simulink model "SHY4_S2"  (R2023a)
settings: Solver=VariableStepAuto  StartTime=0.0  StopTime=1000  RelTol=1e-3
values from neighbouring files (symbols this model uses):
  coolant_initial_temperature = 293.15    [cathode_subsystem_parameters.m]    (also in thermal_subsystem_parameters.m)
  coolant_tube_D = 0.05    [cathode_subsystem_parameters.m]    (also in thermal_subsystem_parameters.m)
  Hydrowell_VTS =     [Hydrowell_values_VLV.mat]
undefined symbols (not defined in the file or in its folder): sigbuilder_block, stack
libraries: fl_lib x135, nesl_utility x104, SimscapeFluids_lib x15, slpidlib x5, simulink x1
(part 3 of 8)

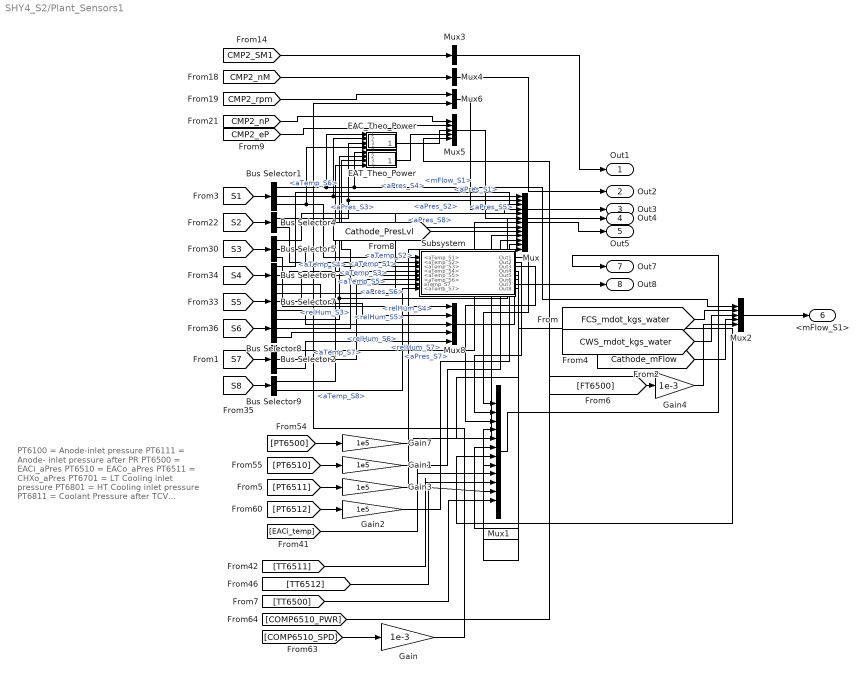
== system SHY4_S2/Plant_Sensors1 ==
  note: PT6100 = Anode-inlet pressure
      | PT6111 = Anode- inlet pressure after PR
      | PT6500 = EACi_aPres
      | PT6510 = EACo_aPres
      | PT6511 = CHXo_aPres
      | PT6701 = LT Cooling inlet pressure
      | PT6801 = HT Cooling inlet pressure
      | PT6811 = Coolant Pressure after TCV
      | PT6114 = FCS H2 inlet pressure
      | PT6512 = FCS O2 inlet Pressure
      | PT6812 = FCS Coolant inlet pressure
      |
      | TT6100 = Anode- inlet Temperature
      | TT6111 = Anode- after Temperature
      | TT6500 = EACi_Temp
      | TT6510 = EACo_Temp
      | TT6701 = LT Cooling inlet Temperature
      | TT6801 = HT Cooling inlet Temperature
      | TT6811 = Coolant Temperature after TCV
      | TT6114 = FCS H2 inlet Temperature
      | TT6512 = FCS O2 inlet Temperature
      | TT6812 = FCS Coolant inlet Temperature
  Bus Selector1 : BusSelector  OutputSignals=mFlow_S1,aPres_S1,aTemp_S1
  Bus Selector2 : BusSelector  OutputSignals=aPres_S7,aTemp_S7,relHum_S7
  Bus Selector4 : BusSelector  OutputSignals=aPres_S2,aTemp_S2
  Bus Selector5 : BusSelector  OutputSignals=aPres_S3,aTemp_S3,relHum_S3
  Bus Selector6 : BusSelector  OutputSignals=aPres_S4,aTemp_S4,relHum_S4
  Bus Selector7 : BusSelector  OutputSignals=aPres_S5,aTemp_S5,relHum_S5
  Bus Selector8 : BusSelector  OutputSignals=aPres_S6,aTemp_S6,relHum_S6
  Bus Selector9 : BusSelector  OutputSignals=aPres_S8,aTemp_S8
  EAC_Theo_Power : Subsystem
  EAT_Theo_Power : Subsystem
  Gain : Gain  Gain=1e-3
  Gain{1..3,7} (4 alike) : Gain  Gain=1e5
  Gain4 : Gain  Gain=1e-3
  Mux : Mux  Inputs=13
  Mux1 : Mux  Inputs=12
  Mux2 : Mux  Inputs=5
  Mux3 : Mux  Inputs=1
  Mux4 : Mux  Inputs=1
  Mux5 : Mux  Inputs=5
  Mux6 : Mux  Inputs=2
  Mux8 : Mux  Inputs=5
  Subsystem : Subsystem
  Out1 : Outport
  Out2 : Outport  Port=2
  Out3 : Outport  Port=3
  Out4 : Outport  Port=4
  Out5 : Outport  Port=5
  <mFlow_S1> : Outport  Port=6
  Out7 : Outport  Port=7
  Out8 : Outport  Port=8
  wires:
  [CMP2_eP] -> Mux5/2
  [CMP2_nP] -> Mux5/1
  Mux3/1 -> Out1/1
  [S8] -> Bus Selector9/1
  [CMP2_SM1] -> Mux3/1
  Bus Selector7/3 -> Mux8/3  "<relHum_S5>"
  Bus Selector9/1 -> EAT_Theo_Power/4(<aPres_S7>), Mux/8  "<aPres_S8>"
  Bus Selector4/1 -> EAC_Theo_Power/3(<aPres_S2>), Mux/2  "<aPres_S2>"
  [CMP2_rpm] -> Mux6/1
  [CMP2_nM] -> Mux4/1
  Bus Selector6/1 -> Mux/4  "<aPres_S4>"
  [S5] -> Bus Selector7/1
  Mux/1 -> Out5/1
  Bus Selector5/3 -> Mux8/1  "<relHum_S3>"
  Bus Selector5/1 -> Mux/3  "<aPres_S3>"
  [S4] -> Bus Selector6/1
  Mux6/1 -> Out3/1
  [S3] -> Bus Selector5/1
  Bus Selector1/1 -> Mux2/1, EAT_Theo_Power/1(<mFlow_S1>), EAC_Theo_Power/1(<mFlow_S1>)  "<mFlow_S1>"
  Bus Selector7/1 -> Mux/5  "<aPres_S5>"
  Bus Selector8/1 -> EAT_Theo_Power/2(<aPres_S6>), Mux/6  "<aPres_S6>"
  [S1] -> Bus Selector1/1
  [Cathode_PresLvl] -> Mux/9
  Mux5/1 -> Out4/1
  Bus Selector6/3 -> Mux8/2  "<relHum_S4>"
  Bus Selector8/3 -> Mux8/4  "<relHum_S6>"
  [S6] -> Bus Selector8/1
  Bus Selector1/2 -> Mux/1, EAC_Theo_Power/2(<aPres_S1>)  "<aPres_S1>"
  [S2] -> Bus Selector4/1
  Mux4/1 -> Out2/1
  Mux1/1 -> Out7/1
  Mux8/1 -> Out8/1
  Bus Selector1/3 -> EAC_Theo_Power/4(<aTemp_S1>), Subsystem/1(<aTemp_S1>)  "<aTemp_S1>"
  Bus Selector4/2 -> Subsystem/2(<aTemp_S2>)  "<aTemp_S2>"
  Bus Selector5/2 -> Subsystem/3(<aTemp_S3>)  "<aTemp_S3>"
  Bus Selector6/2 -> Subsystem/4(<aTemp_S4>)  "<aTemp_S4>"
  Bus Selector7/2 -> Subsystem/5(<aTemp_S5>)  "<aTemp_S5>"
  Bus Selector8/2 -> EAT_Theo_Power/3(<aTemp_S6>), Subsystem/6(<aTemp_S6>)  "<aTemp_S6>"
  Bus Selector9/2 -> Subsystem/8(<aTemp_S7>)  "<aTemp_S8>"
  Subsystem/1(Out1) -> Mux1/1
  Subsystem/2(Out2) -> Mux1/2
  Subsystem/3(Out3) -> Mux1/3
  Subsystem/4(Out4) -> Mux1/4
  Subsystem/5(Out5) -> Mux1/5
  Subsystem/6(Out6) -> Mux1/6
  Subsystem/7(Out7) -> Mux1/7
  EAC_Theo_Power/1(Out1) -> Mux5/3
  EAT_Theo_Power/1(Out1) -> Mux5/4
  [S7] -> Bus Selector2/1
  Bus Selector2/2 -> Subsystem/7(aTemp_S7)  "<aTemp_S7>"
  Subsystem/8(Out8) -> Mux1/8
  Bus Selector2/1 -> Mux/7  "<aPres_S7>"
  Bus Selector2/3 -> Mux8/5  "<relHum_S7>"
  [FCS_mdot_kgs_water] -> Mux2/2
  Mux2/1 -> <mFlow_S1>/1
  [Cathode_mFlow] -> Mux2/4
  [CWS_mdot_kgs_water] -> Mux2/3
  Gain1/1 -> Mux/11
  [COMP6510_SPD] -> Gain/1
  Gain2/1 -> Mux/12
  [PT6500] -> Gain7/1
  [EACi_temp] -> Mux1/9
  [TT6512] -> Mux1/11
  [PT6512] -> Gain2/1
  [TT6500] -> Mux1/12
  [TT6511] -> Mux1/10
  [COMP6510_PWR] -> Mux5/5
  [PT6510] -> Gain1/1
  Gain7/1 -> Mux/10
  Gain/1 -> Mux6/2
  [PT6511] -> Gain3/1
  Gain3/1 -> Mux/13
  [FT6500] -> Gain4/1
  Gain4/1 -> Mux2/5

== system SHY4_S2/Subsystem ==
  <aTemp_S4> : Inport
  Constant : Constant  Value=273.15
  Minus : Sum  Inputs=+-
  Out1 : Outport
  wires:
  Constant/1 -> Minus/2
  <aTemp_S4>/1 -> Minus/1
  Minus/1 -> Out1/1

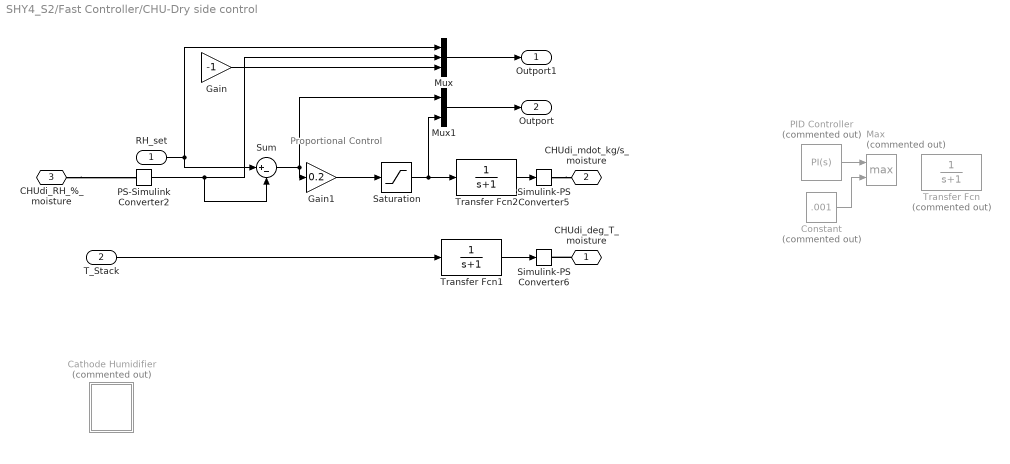
== system SHY4_S2/Fast Controller/CHU-Dry side control ==
  note: Proportional Control
  RH_set : Inport
  T_Stack : Inport  Port=2
  Cathode Humidifier : Subsystem  Tag=PublishSubsystem  Commented=on
  Constant : Constant  Commented=on  Value=.001
  Gain : Gain  Gain=-1
  Gain1 : Gain  Gain=0.2
  Max : MinMax  Commented=on  Function=max  Inputs=2
  Mux : Mux  Inputs=3
  Mux1 : Mux  Inputs=2
  PID Controller : slpidlib/PID Controller  Commented=on  Controller=PI  Form=Parallel  TimeDomain=Continuous-time  UseExternalTs=off  SampleTime=-1  IntegratorMethod=Forward Euler  FilterMethod=Forward Euler  ControllerParametersSource=internal  P=1  I=1  UseKiTs=off  D=0  N=100  UseFilter=on  TunerSelectOption=Transfer Function Based (PID Tuner App)  InitialConditionSource=internal  InitialConditionForIntegrator=0  InitialConditionForFilter=0  DifferentiatorICPrevScaledInput=0  ExternalReset=none  TrackingMode=off  Kt=1  LimitOutput=off  SatLimitsSource=internal  UpperSaturationLimit=inf  LowerSaturationLimit=-inf  LinearizeAsGain=on  AntiWindupMode=none  Kb=1  LimitIntegrator=off  UpperIntegratorSaturationLimit=inf  LowerIntegratorSaturationLimit=-inf  POutMin=[]  POutMax=[]  IOutMin=[]  IOutMax=[]  DOutMin=[]  DOutMax=[]  NOutMin=[]  NOutMax=[]  SumOutMin=[]  SumOutMax=[]  SaturationOutMin=[]  SaturationOutMax=[]  PParamMin=[]  PParamMax=[]  IParamMin=[]  IParamMax=[]  DParamMin=[]  DParamMax=[]  NParamMin=[]  NParamMax=[]  KbParamMin=[]  KbParamMax=[]  KtParamMin=[]  KtParamMax=[]  KbOutMin=[]  KbOutMax=[]  KtOutMin=[]  KtOutMax=[]  IntegratorOutMin=[]  IntegratorOutMax=[]  FilterOutMin=[]  FilterOutMax=[]  SumI1OutMin=[]  SumI1OutMax=[]  SumI2OutMin=[]  SumI2OutMax=[]  SumI3OutMin=[]  SumI3OutMax=[]  SumI4OutMin=[]  SumI4OutMax=[]  SumDOutMin=[]  SumDOutMax=[]  DifferentiatorOutMin=[]  DifferentiatorOutMax=[]  FilterDiffOutCoefMin=[]  FilterDiffOutCoefMax=[]  ReciprocalOutMin=[]  ReciprocalOutMax=[]  SumDenOutMin=[]  SumDenOutMax=[]  SumNumOutMin=[]  SumNumOutMax=[]  DivideOutMin=[]  DivideOutMax=[]  UdiffTsProdOutMin=[]  UdiffTsProdOutMax=[]  NTsProdOutMin=[]  NTsProdOutMax=[]  UintegralTsProdOutMin=[]  UintegralTsProdOutMax=[]  UngainTsProdOutMin=[]  UngainTsProdOutMax=[]  ClampingZeroOutDataTypeStr=Inherit: Inherit via back propagation  ClampingZeroOutMin=[]  ClampingZeroOutMax=[]  FilterDenConstantOutDataTypeStr=Inherit: Inherit via back propagation  FilterDenConstantOutMin=[]  FilterDenConstantOutMax=[]  PCopyOutDataTypeStr=Inherit: Inherit via back propagation  PCopyOutMin=[]  PCopyOutMax=[]  NCopyOutDataTypeStr=Inherit: Inherit via back propagation  NCopyOutMin=[]  NCopyOutMax=[]  IntegratorContinuousStateAttributes=''  IntegratorStateMustResolveToSignalObject=off  IntegratorRTWStateStorageClass=Auto  FilterContinuousStateAttributes=''  FilterStateMustResolveToSignalObject=off  FilterRTWStateStorageClass=Auto  ParallelPVariant=InternalParameters  IdealPVariant=Disabled  IVariant=InternalParameters  DVariant=Disabled  IntegratorVariant=Continuous  SatVariant=Disabled  AWVariant=Passthrough  PCopyVariant=Disabled  TRVariant=Disabled  FdbkBlocksVariant=Forward  IdealPFdbkVariant=Disabled  SatFdbkVariant=Disabled  DerivativeFilterVariant=Disabled  NVariant=Disabled  NCopyVariant=Disabled_SignalSpec  FilterICVariant=Disabled  IntegratorICVariant=InternalICs  ExternalResetVariant=Disabled  TRSumVariant=Passthrough  SumFdbkVariant=Disabled  SumVariant=Sum_PI  TsampFilterVariant=InternalTs  TsampNgainVariant=Passthrough  TsampIntegralVariant=Disabled_SignalSpec  ExternalSaturationOutDataTypeStr=Inherit: Same as second input
  PS-Simulink Converter2 : nesl_utility/PS-Simulink Converter  PhysicalDomain=network_engine_domain  SubClassName=ps_output  LeftPortType=input  RightPortType=output  PseudoPeriodic=off  Frequencies=[]  VectorFormat=1-D array  Unit=1  AffineConversion=off
  Saturation : Saturate  UpperLimit=inf  LowerLimit=0  ZeroCross=off
  Simulink-PS Converter5 : nesl_utility/Simulink-PS Converter  PhysicalDomain=network_engine_domain  SubClassName=ps_input  LeftPortType=input  RightPortType=output  PseudoPeriodic=off  Frequencies=[]  NoiseDistribution=none  NoiseParameters=[]  Unit=kg/s  AffineConversion=off  FilteringAndDerivatives=provide  SimscapeFilterOrder=1  InputFilterTimeConstant=0.001  UdotUserProvided=0
  Simulink-PS Converter6 : nesl_utility/Simulink-PS Converter  PhysicalDomain=network_engine_domain  SubClassName=ps_input  LeftPortType=input  RightPortType=output  PseudoPeriodic=off  Frequencies=[]  NoiseDistribution=none  NoiseParameters=[]  Unit=degC  AffineConversion=on  FilteringAndDerivatives=provide  SimscapeFilterOrder=1  InputFilterTimeConstant=0.001  UdotUserProvided=0
  Sum : Sum  Inputs=|+-
  Transfer Fcn : TransferFcn  Commented=on  Denominator=[1 1]
  Transfer Fcn1 : TransferFcn  Denominator=[1 1]
  Transfer Fcn2 : TransferFcn  Denominator=[1 1]
  CHUdi_deg_T_moisture : PMIOPort  Side=Right
  CHUdi_mdot_kg/s_moisture : PMIOPort  Port=2  Side=Right
  CHUdi_RH_%_moisture : PMIOPort  Port=3  Side=Right
  Outport1 : Outport
  Outport : Outport  Port=2
  wires:
  Transfer Fcn2/1 -> Simulink-PS Converter5/1
  T_Stack/1 -> Transfer Fcn1/1
  Transfer Fcn1/1 -> Simulink-PS Converter6/1
  Constant/1 -> Max/2
  PID Controller/1 -> Max/1
  PS-Simulink Converter2/1 -> Mux/2, Sum/2
  RH_set/1 -> Mux/1, Sum/1
  Mux/1 -> Outport1/1
  Mux1/1 -> Outport/1
  Gain/1 -> Mux/3
  Gain1/1 -> Saturation/1
  Saturation/1 -> Mux1/2, Transfer Fcn2/1
  Sum/1 -> Gain1/1, Mux1/1
  connections:
  Simulink-PS Converter5/RConn1 -- CHUdi_mdot_kg/s_moisture/RConn1
  CHUdi_deg_T_moisture/RConn1 -- Simulink-PS Converter6/RConn1
  CHUdi_RH_%_moisture/RConn1 -- PS-Simulink Converter2/LConn1

== system SHY4_S2/Fast Controller/CHU-wet side control ==
  <aTemp_S5> : Inport
  RH_set : Inport  Port=2
  <RH_S5> : Inport  Port=3
  Constant : Constant  Value=-.2
  Mux : Mux  Inputs=2
  Mux1 : Mux  Inputs=2
  Saturation : Saturate  Commented=on  UpperLimit=inf  LowerLimit=-.1  ZeroCross=off
  Simulink-PS Converter : nesl_utility/Simulink-PS Converter  PhysicalDomain=network_engine_domain  SubClassName=ps_input  LeftPortType=input  RightPortType=output  PseudoPeriodic=off  Frequencies=[]  NoiseDistribution=none  NoiseParameters=[]  Unit=kg/s  AffineConversion=off  FilteringAndDerivatives=provide  SimscapeFilterOrder=1  InputFilterTimeConstant=0.001  UdotUserProvided=0
  Simulink-PS Converter2 : nesl_utility/Simulink-PS Converter  PhysicalDomain=network_engine_domain  SubClassName=ps_input  LeftPortType=input  RightPortType=output  PseudoPeriodic=off  Frequencies=[]  NoiseDistribution=none  NoiseParameters=[]  Unit=degC  AffineConversion=on  FilteringAndDerivatives=provide  SimscapeFilterOrder=1  InputFilterTimeConstant=0.001  UdotUserProvided=0
  Sum : Sum  Commented=on  Inputs=|+-
  Transfer Fcn : TransferFcn  Commented=on  Denominator=[3 1]
  Transfer Fcn1 : TransferFcn  Denominator=[1 1]
  CHUwi_mdot_kg/s_moisture : PMIOPort  Side=Right
  CHUwi_T_degC_moisture : PMIOPort  Port=2  Side=Right
  Outport : Outport
  Outport1 : Outport  Port=2
  wires:
  Transfer Fcn1/1 -> Simulink-PS Converter2/1
  <aTemp_S5>/1 -> Transfer Fcn1/1
  Transfer Fcn/1 -> Mux1/2
  <RH_S5>/1 -> Mux/2, Sum/2
  Mux1/1 -> Outport1/1
  Saturation/1 -> Mux1/1, Transfer Fcn/1
  Mux/1 -> Outport/1
  RH_set/1 -> Mux/1, Sum/1
  Sum/1 -> Saturation/1
  Constant/1 -> Simulink-PS Converter/1
  connections:
  Simulink-PS Converter/RConn1 -- CHUwi_T_degC_moisture/RConn1
  CHUwi_mdot_kg/s_moisture/RConn1 -- Simulink-PS Converter2/RConn1

== system SHY4_S2/Fast Controller/CWS-controller ==
  <aTemp_S5> : Inport
  RH_set : Inport  Port=2
  CWSo_RH_%_moisture : Inport  Port=3
  Mux : Mux  Inputs=2
  Mux1 : Mux  Inputs=2
  PID Controller : slpidlib/PID Controller  Controller=PI  Form=Parallel  TimeDomain=Continuous-time  UseExternalTs=off  SampleTime=-1  IntegratorMethod=Forward Euler  FilterMethod=Forward Euler  ControllerParametersSource=internal  P=1  I=1  UseKiTs=off  D=0  N=100  UseFilter=on  TunerSelectOption=Transfer Function Based (PID Tuner App)  InitialConditionSource=internal  InitialConditionForIntegrator=0  InitialConditionForFilter=0  DifferentiatorICPrevScaledInput=0  ExternalReset=none  TrackingMode=off  Kt=1  LimitOutput=on  SatLimitsSource=internal  UpperSaturationLimit=.2  LowerSaturationLimit=-.2  LinearizeAsGain=off  AntiWindupMode=none  Kb=1  LimitIntegrator=off  UpperIntegratorSaturationLimit=inf  LowerIntegratorSaturationLimit=-inf  POutMin=[]  POutMax=[]  IOutMin=[]  IOutMax=[]  DOutMin=[]  DOutMax=[]  NOutMin=[]  NOutMax=[]  SumOutMin=[]  SumOutMax=[]  SaturationOutMin=[]  SaturationOutMax=[]  PParamMin=[]  PParamMax=[]  IParamMin=[]  IParamMax=[]  DParamMin=[]  DParamMax=[]  NParamMin=[]  NParamMax=[]  KbParamMin=[]  KbParamMax=[]  KtParamMin=[]  KtParamMax=[]  KbOutMin=[]  KbOutMax=[]  KtOutMin=[]  KtOutMax=[]  IntegratorOutMin=[]  IntegratorOutMax=[]  FilterOutMin=[]  FilterOutMax=[]  SumI1OutMin=[]  SumI1OutMax=[]  SumI2OutMin=[]  SumI2OutMax=[]  SumI3OutMin=[]  SumI3OutMax=[]  SumI4OutMin=[]  SumI4OutMax=[]  SumDOutMin=[]  SumDOutMax=[]  DifferentiatorOutMin=[]  DifferentiatorOutMax=[]  FilterDiffOutCoefMin=[]  FilterDiffOutCoefMax=[]  ReciprocalOutMin=[]  ReciprocalOutMax=[]  SumDenOutMin=[]  SumDenOutMax=[]  SumNumOutMin=[]  SumNumOutMax=[]  DivideOutMin=[]  DivideOutMax=[]  UdiffTsProdOutMin=[]  UdiffTsProdOutMax=[]  NTsProdOutMin=[]  NTsProdOutMax=[]  UintegralTsProdOutMin=[]  UintegralTsProdOutMax=[]  UngainTsProdOutMin=[]  UngainTsProdOutMax=[]  ClampingZeroOutDataTypeStr=Inherit: Inherit via back propagation  ClampingZeroOutMin=[]  ClampingZeroOutMax=[]  FilterDenConstantOutDataTypeStr=Inherit: Inherit via back propagation  FilterDenConstantOutMin=[]  FilterDenConstantOutMax=[]  PCopyOutDataTypeStr=Inherit: Inherit via back propagation  PCopyOutMin=[]  PCopyOutMax=[]  NCopyOutDataTypeStr=Inherit: Inherit via back propagation  NCopyOutMin=[]  NCopyOutMax=[]  IntegratorContinuousStateAttributes=''  IntegratorStateMustResolveToSignalObject=off  IntegratorRTWStateStorageClass=Auto  FilterContinuousStateAttributes=''  FilterStateMustResolveToSignalObject=off  FilterRTWStateStorageClass=Auto  ParallelPVariant=InternalParameters  IdealPVariant=Disabled  IVariant=InternalParameters  DVariant=Disabled  IntegratorVariant=Continuous  SatVariant=Enabled  AWVariant=Passthrough  PCopyVariant=Disabled  TRVariant=Disabled  FdbkBlocksVariant=Forward  IdealPFdbkVariant=Disabled  SatFdbkVariant=Disabled  DerivativeFilterVariant=Disabled  NVariant=Disabled  NCopyVariant=Disabled_SignalSpec  FilterICVariant=Disabled  IntegratorICVariant=InternalICs  ExternalResetVariant=Disabled  TRSumVariant=Passthrough  SumFdbkVariant=Disabled  SumVariant=Sum_PI  TsampFilterVariant=InternalTs  TsampNgainVariant=Passthrough  TsampIntegralVariant=Disabled_SignalSpec  ExternalSaturationOutDataTypeStr=Inherit: Same as second input
  Simulink-PS Converter5 : nesl_utility/Simulink-PS Converter  PhysicalDomain=network_engine_domain  SubClassName=ps_input  LeftPortType=input  RightPortType=output  PseudoPeriodic=off  Frequencies=[]  NoiseDistribution=none  NoiseParameters=[]  Unit=kg/s  AffineConversion=off  FilteringAndDerivatives=provide  SimscapeFilterOrder=1  InputFilterTimeConstant=0.001  UdotUserProvided=0
  Sum : Sum  Inputs=|+-
  Transfer Fcn : TransferFcn  Denominator=[4 1]
  CWS_mdot_kg/s_moisture : PMIOPort  Side=Right
  Outport : Outport
  Outport1 : Outport  Port=2
  wires:
  Sum/1 -> PID Controller/1
  Transfer Fcn/1 -> Simulink-PS Converter5/1, Mux1/2
  CWSo_RH_%_moisture/1 -> Mux/2, Sum/2
  Mux1/1 -> Outport1/1
  PID Controller/1 -> Mux1/1, Transfer Fcn/1
  Mux/1 -> Outport/1
  RH_set/1 -> Mux/1, Sum/1
  connections:
  Simulink-PS Converter5/RConn1 -- CWS_mdot_kg/s_moisture/RConn1

== system SHY4_S2/Fast Controller/Compressor Controller  ==
  set : Inport
  meas : Inport  Port=2
  Gain : Gain  Gain=450
  Mux10 : Mux  Inputs=2
  Mux11 : Mux  Inputs=2
  PID_CMP : slpidlib/PID Controller  Controller=PID  Form=Parallel  TimeDomain=Continuous-time  UseExternalTs=off  SampleTime=-1  IntegratorMethod=Forward Euler  FilterMethod=Forward Euler  ControllerParametersSource=internal  P=6  I=1.5  UseKiTs=off  D=-4.2  N=1.81801523459338  UseFilter=on  TunerSelectOption=Transfer Function Based (PID Tuner App)  InitialConditionSource=internal  InitialConditionForIntegrator=0  InitialConditionForFilter=0  DifferentiatorICPrevScaledInput=0  ExternalReset=none  TrackingMode=off  Kt=1  LimitOutput=on  SatLimitsSource=internal  UpperSaturationLimit=1  LowerSaturationLimit=0  LinearizeAsGain=off  AntiWindupMode=clamping  Kb=1  LimitIntegrator=off  UpperIntegratorSaturationLimit=inf  LowerIntegratorSaturationLimit=-inf  POutMin=[]  POutMax=[]  IOutMin=[]  IOutMax=[]  DOutMin=[]  DOutMax=[]  NOutMin=[]  NOutMax=[]  SumOutMin=[]  SumOutMax=[]  SaturationOutMin=[]  SaturationOutMax=[]  PParamMin=[]  PParamMax=[]  IParamMin=[]  IParamMax=[]  DParamMin=[]  DParamMax=[]  NParamMin=[]  NParamMax=[]  KbParamMin=[]  KbParamMax=[]  KtParamMin=[]  KtParamMax=[]  KbOutMin=[]  KbOutMax=[]  KtOutMin=[]  KtOutMax=[]  IntegratorOutMin=[]  IntegratorOutMax=[]  FilterOutMin=[]  FilterOutMax=[]  SumI1OutMin=[]  SumI1OutMax=[]  SumI2OutMin=[]  SumI2OutMax=[]  SumI3OutMin=[]  SumI3OutMax=[]  SumI4OutMin=[]  SumI4OutMax=[]  SumDOutMin=[]  SumDOutMax=[]  DifferentiatorOutMin=[]  DifferentiatorOutMax=[]  FilterDiffOutCoefMin=[]  FilterDiffOutCoefMax=[]  ReciprocalOutMin=[]  ReciprocalOutMax=[]  SumDenOutMin=[]  SumDenOutMax=[]  SumNumOutMin=[]  SumNumOutMax=[]  DivideOutMin=[]  DivideOutMax=[]  UdiffTsProdOutMin=[]  UdiffTsProdOutMax=[]  NTsProdOutMin=[]  NTsProdOutMax=[]  UintegralTsProdOutMin=[]  UintegralTsProdOutMax=[]  UngainTsProdOutMin=[]  UngainTsProdOutMax=[]  ClampingZeroOutDataTypeStr=Inherit: Inherit via back propagation  ClampingZeroOutMin=[]  ClampingZeroOutMax=[]  FilterDenConstantOutDataTypeStr=Inherit: Inherit via back propagation  FilterDenConstantOutMin=[]  FilterDenConstantOutMax=[]  PCopyOutDataTypeStr=Inherit: Inherit via back propagation  PCopyOutMin=[]  PCopyOutMax=[]  NCopyOutDataTypeStr=Inherit: Inherit via back propagation  NCopyOutMin=[]  NCopyOutMax=[]  IntegratorContinuousStateAttributes=''  IntegratorStateMustResolveToSignalObject=off  IntegratorRTWStateStorageClass=Auto  FilterContinuousStateAttributes=''  FilterStateMustResolveToSignalObject=off  FilterRTWStateStorageClass=Auto  ParallelPVariant=InternalParameters  IdealPVariant=Disabled  IVariant=InternalParameters  DVariant=InternalParameters  IntegratorVariant=Continuous  SatVariant=Enabled  AWVariant=ContClampingParallel  PCopyVariant=Disabled  TRVariant=Disabled  FdbkBlocksVariant=Forward  IdealPFdbkVariant=Disabled  SatFdbkVariant=Disabled  DerivativeFilterVariant=ContFilter  NVariant=InternalParameters  NCopyVariant=Disabled  FilterICVariant=InternalICsFilter  IntegratorICVariant=InternalICs  ExternalResetVariant=Disabled  TRSumVariant=Passthrough  SumFdbkVariant=Disabled  SumVariant=Sum_PID  TsampFilterVariant=InternalTs  TsampNgainVariant=Passthrough  TsampIntegralVariant=Disabled_SignalSpec  ExternalSaturationOutDataTypeStr=Inherit: Same as second input
  Plus1 : Sum  Inputs=-+
  Transfer Fcn1 : TransferFcn  Denominator=[3 1]  ParameterTunability=Optimized
  Out1 : Outport
  Out2 : Outport  Port=2
  Out3 : Outport  Port=3
  wires:
  meas/1 -> Mux10/2, Plus1/1
  Mux11/1 -> Out3/1
  Plus1/1 -> PID_CMP/1  "ctrl_error"
  Mux10/1 -> Out2/1
  set/1 -> Mux10/1, Plus1/2
  Gain/1 -> Out1/1
  PID_CMP/1 -> Transfer Fcn1/1, Mux11/2  "PID_o"
  Transfer Fcn1/1 -> Gain/1, Mux11/1  "com2_omega"

== system SHY4_S2/Fast Controller/Temperature Control ==
  T_set : Inport
  In2 : Inport  Port=2
  Max Flow2 : fl_lib/Physical Signals/Functions/PS Gain  gain=2
  Mux : Mux  Inputs=2
  Mux1 : Mux  Inputs=2
  PID Controller : slpidlib/PID Controller  Controller=PI  Form=Ideal  TimeDomain=Continuous-time  UseExternalTs=off  SampleTime=-1  IntegratorMethod=Forward Euler  FilterMethod=Forward Euler  ControllerParametersSource=internal  P=1  I=0.1  UseKiTs=off  D=0  N=100  UseFilter=on  TunerSelectOption=Frequency Response Based  ZeroCross=off  InitialConditionSource=internal  InitialConditionForIntegrator=0  InitialConditionForFilter=0  DifferentiatorICPrevScaledInput=0  ExternalReset=none  TrackingMode=off  Kt=1  LimitOutput=on  SatLimitsSource=internal  UpperSaturationLimit=1  LowerSaturationLimit=0  LinearizeAsGain=on  AntiWindupMode=clamping  Kb=1  LimitIntegrator=off  UpperIntegratorSaturationLimit=inf  LowerIntegratorSaturationLimit=-inf  POutMin=[]  POutMax=[]  IOutMin=[]  IOutMax=[]  DOutMin=[]  DOutMax=[]  NOutMin=[]  NOutMax=[]  SumOutMin=[]  SumOutMax=[]  SaturationOutMin=[]  SaturationOutMax=[]  PParamMin=[]  PParamMax=[]  IParamMin=[]  IParamMax=[]  DParamMin=[]  DParamMax=[]  NParamMin=[]  NParamMax=[]  KbParamMin=[]  KbParamMax=[]  KtParamMin=[]  KtParamMax=[]  KbOutMin=[]  KbOutMax=[]  KtOutMin=[]  KtOutMax=[]  IntegratorOutMin=[]  IntegratorOutMax=[]  FilterOutMin=[]  FilterOutMax=[]  SumI1OutMin=[]  SumI1OutMax=[]  SumI2OutMin=[]  SumI2OutMax=[]  SumI3OutMin=[]  SumI3OutMax=[]  SumI4OutMin=[]  SumI4OutMax=[]  SumDOutMin=[]  SumDOutMax=[]  DifferentiatorOutMin=[]  DifferentiatorOutMax=[]  FilterDiffOutCoefMin=[]  FilterDiffOutCoefMax=[]  ReciprocalOutMin=[]  ReciprocalOutMax=[]  SumDenOutMin=[]  SumDenOutMax=[]  SumNumOutMin=[]  SumNumOutMax=[]  DivideOutMin=[]  DivideOutMax=[]  UdiffTsProdOutMin=[]  UdiffTsProdOutMax=[]  NTsProdOutMin=[]  NTsProdOutMax=[]  UintegralTsProdOutMin=[]  UintegralTsProdOutMax=[]  UngainTsProdOutMin=[]  UngainTsProdOutMax=[]  ClampingZeroOutDataTypeStr=Inherit: Inherit via back propagation  ClampingZeroOutMin=[]  ClampingZeroOutMax=[]  FilterDenConstantOutDataTypeStr=Inherit: Inherit via back propagation  FilterDenConstantOutMin=[]  FilterDenConstantOutMax=[]  PCopyOutDataTypeStr=Inherit: Inherit via back propagation  PCopyOutMin=[]  PCopyOutMax=[]  NCopyOutDataTypeStr=Inherit: Inherit via back propagation  NCopyOutMin=[]  NCopyOutMax=[]  IntegratorContinuousStateAttributes=''  IntegratorStateMustResolveToSignalObject=off  IntegratorRTWStateStorageClass=Auto  FilterContinuousStateAttributes=''  FilterStateMustResolveToSignalObject=off  FilterRTWStateStorageClass=Auto  ParallelPVariant=Passthrough  IdealPVariant=InternalParameters  IVariant=InternalParameters  DVariant=Disabled  IntegratorVariant=Continuous  SatVariant=Enabled  AWVariant=ContClampingIdeal  PCopyVariant=InternalParamsIdeal  TRVariant=Disabled  FdbkBlocksVariant=Forward  IdealPFdbkVariant=Disabled  SatFdbkVariant=Disabled  DerivativeFilterVariant=Disabled  NVariant=Disabled  NCopyVariant=Disabled_SignalSpec  FilterICVariant=Disabled  IntegratorICVariant=InternalICs  ExternalResetVariant=Disabled  TRSumVariant=Passthrough  SumFdbkVariant=Disabled  SumVariant=Sum_PI  TsampFilterVariant=InternalTs  TsampNgainVariant=Passthrough  TsampIntegralVariant=Disabled_SignalSpec  ExternalSaturationOutDataTypeStr=Inherit: Same as second input
  Simulink-PS Converter3 : nesl_utility/Simulink-PS Converter  PhysicalDomain=network_engine_domain  SubClassName=ps_input  LeftPortType=input  RightPortType=output  PseudoPeriodic=off  Frequencies=[]  NoiseDistribution=none  NoiseParameters=[]  Unit=1  AffineConversion=off  FilteringAndDerivatives=provide  SimscapeFilterOrder=1  InputFilterTimeConstant=0.001  UdotUserProvided=0
  Sum : Sum  Inputs=+-
  Transfer Fcn : TransferFcn  Denominator=[2 1]
  Connection Port : PMIOPort  Side=Right
  Outport : Outport
  Outport1 : Outport  Port=2
  wires:
  Transfer Fcn/1 -> Simulink-PS Converter3/1, Mux1/2
  T_set/1 -> Mux/1, Sum/2
  Sum/1 -> PID Controller/1
  PID Controller/1 -> Mux1/1, Transfer Fcn/1
  Mux/1 -> Outport/1
  Mux1/1 -> Outport1/1
  In2/1 -> Sum/1, Mux/2
  connections:
  Max Flow2/RConn1 -- Connection Port/RConn1
  Simulink-PS Converter3/RConn1 -- Max Flow2/LConn1

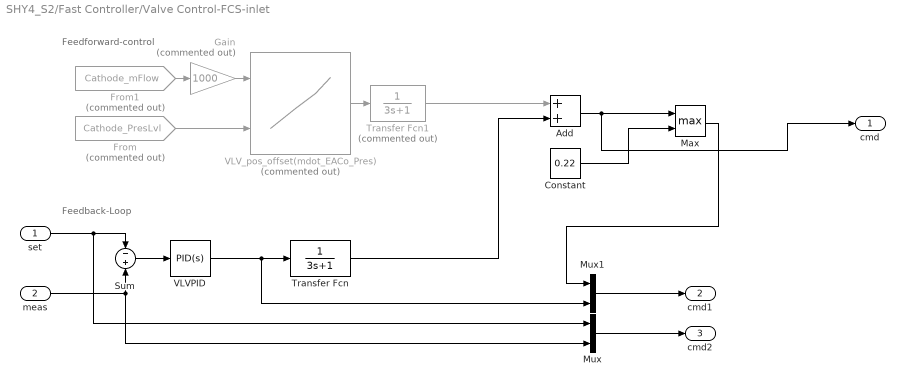
== system SHY4_S2/Fast Controller/Valve Control-FCS-inlet ==
  note: Feedback-Loop
  note: Feedforward-control
  set : Inport
  meas : Inport  Port=2
  Add : Sum
  Constant : Constant  Value=0.22
  From : From  Commented=on  GotoTag=Cathode_PresLvl  TagVisibility=global
  From1 : From  Commented=on  GotoTag=Cathode_mFlow  TagVisibility=global
  Gain : Gain  Commented=on  Gain=1000
  Max : MinMax  Function=max  Inputs=2
  Mux : Mux  Inputs=2
  Mux1 : Mux  Inputs=2
  Sum : Sum  Inputs=-+
  Transfer Fcn : TransferFcn  Denominator=[3 1]
  Transfer Fcn1 : TransferFcn  Commented=on  Denominator=[3 1]
  VLVPID : slpidlib/PID Controller  Controller=PID  Form=Parallel  TimeDomain=Continuous-time  UseExternalTs=off  SampleTime=-1  IntegratorMethod=Forward Euler  FilterMethod=Forward Euler  ControllerParametersSource=internal  P=0.000922965512409213  I=0.000345236154843816  UseKiTs=off  D=0.000211713179859515  N=2.31640255659242  UseFilter=on  TunerSelectOption=Transfer Function Based (PID Tuner App)  InitialConditionSource=internal  InitialConditionForIntegrator=0  InitialConditionForFilter=0  DifferentiatorICPrevScaledInput=0  ExternalReset=none  TrackingMode=off  Kt=1  LimitOutput=on  SatLimitsSource=internal  UpperSaturationLimit=1  LowerSaturationLimit=0  LinearizeAsGain=off  AntiWindupMode=clamping  Kb=1  LimitIntegrator=off  UpperIntegratorSaturationLimit=inf  LowerIntegratorSaturationLimit=.02  POutMin=[]  POutMax=[]  IOutMin=[]  IOutMax=[]  DOutMin=[]  DOutMax=[]  NOutMin=[]  NOutMax=[]  SumOutMin=[]  SumOutMax=[]  SaturationOutMin=[]  SaturationOutMax=[]  PParamMin=[]  PParamMax=[]  IParamMin=[]  IParamMax=[]  DParamMin=[]  DParamMax=[]  NParamMin=[]  NParamMax=[]  KbParamMin=[]  KbParamMax=[]  KtParamMin=[]  KtParamMax=[]  KbOutMin=[]  KbOutMax=[]  KtOutMin=[]  KtOutMax=[]  IntegratorOutMin=[]  IntegratorOutMax=[]  FilterOutMin=[]  FilterOutMax=[]  SumI1OutMin=[]  SumI1OutMax=[]  SumI2OutMin=[]  SumI2OutMax=[]  SumI3OutMin=[]  SumI3OutMax=[]  SumI4OutMin=[]  SumI4OutMax=[]  SumDOutMin=[]  SumDOutMax=[]  DifferentiatorOutMin=[]  DifferentiatorOutMax=[]  FilterDiffOutCoefMin=[]  FilterDiffOutCoefMax=[]  ReciprocalOutMin=[]  ReciprocalOutMax=[]  SumDenOutMin=[]  SumDenOutMax=[]  SumNumOutMin=[]  SumNumOutMax=[]  DivideOutMin=[]  DivideOutMax=[]  UdiffTsProdOutMin=[]  UdiffTsProdOutMax=[]  NTsProdOutMin=[]  NTsProdOutMax=[]  UintegralTsProdOutMin=[]  UintegralTsProdOutMax=[]  UngainTsProdOutMin=[]  UngainTsProdOutMax=[]  ClampingZeroOutDataTypeStr=Inherit: Inherit via back propagation  ClampingZeroOutMin=[]  ClampingZeroOutMax=[]  FilterDenConstantOutDataTypeStr=Inherit: Inherit via back propagation  FilterDenConstantOutMin=[]  FilterDenConstantOutMax=[]  PCopyOutDataTypeStr=Inherit: Inherit via back propagation  PCopyOutMin=[]  PCopyOutMax=[]  NCopyOutDataTypeStr=Inherit: Inherit via back propagation  NCopyOutMin=[]  NCopyOutMax=[]  IntegratorContinuousStateAttributes=''  IntegratorStateMustResolveToSignalObject=off  IntegratorRTWStateStorageClass=Auto  FilterContinuousStateAttributes=''  FilterStateMustResolveToSignalObject=off  FilterRTWStateStorageClass=Auto  ParallelPVariant=InternalParameters  IdealPVariant=Disabled  IVariant=InternalParameters  DVariant=InternalParameters  IntegratorVariant=Continuous  SatVariant=Enabled  AWVariant=ContClampingParallel  PCopyVariant=Disabled  TRVariant=Disabled  FdbkBlocksVariant=Forward  IdealPFdbkVariant=Disabled  SatFdbkVariant=Disabled  DerivativeFilterVariant=ContFilter  NVariant=InternalParameters  NCopyVariant=Disabled  FilterICVariant=InternalICsFilter  IntegratorICVariant=InternalICs  ExternalResetVariant=Disabled  TRSumVariant=Passthrough  SumFdbkVariant=Disabled  SumVariant=Sum_PID  TsampFilterVariant=InternalTs  TsampNgainVariant=Passthrough  TsampIntegralVariant=Disabled_SignalSpec  ExternalSaturationOutDataTypeStr=Inherit: Same as second input
  VLV_pos_offset(mdot_EACo_Pres) : Lookup_n-D  Commented=on  BreakpointsForDimension1=Hydrowell_VTS.mdot_simple  BreakpointsForDimension2=Hydrowell_VTS.pr_simple  Table=Hydrowell_VTS.pr_ETV_position  InternalRulePriority=Speed  RndMeth=Simplest
      settings: InputPortMap=u0,u1
  cmd : Outport
  cmd1 : Outport  Port=2
  cmd2 : Outport  Port=3
  wires:
  set/1 -> Sum/1, Mux/1
  Mux/1 -> cmd2/1
  Mux1/1 -> cmd1/1
  meas/1 -> Mux/2, Sum/2
  Transfer Fcn/1 -> Add/2
  VLVPID/1 -> Mux1/2, Transfer Fcn/1
  Gain/1 -> VLV_pos_offset(mdot_EACo_Pres)/1
  From/1 -> VLV_pos_offset(mdot_EACo_Pres)/2
  VLV_pos_offset(mdot_EACo_Pres)/1 -> Transfer Fcn1/1
  Transfer Fcn1/1 -> Add/1
  Sum/1 -> VLVPID/1
  Add/1 -> cmd/1, Max/1
  From1/1 -> Gain/1
  Constant/1 -> Max/2
  Max/1 -> Mux1/1

== system SHY4_S2/Plant Model H175-Cathode-S1/Coolant Tank1 ==
  Coolant Volume : fl_lib/Thermal Liquid/Elements/Translational Mechanical Converter (TL)  mech_orientation=foundation.enum.MechOrientationTranslational.Positive  displacement_spec=foundation.enum.DisplacementSpec.Calculate  x0=x_init m  interface_area=A m^2  dead_volume=A * 0.005 m^3  environment_spec=foundation.enum.pressure_spec.atmospheric  environment_pressure=0.101325 MPa  dynamic_compressibility=simscape.enum.onoff.off  p0=env_p MPa  T0=30 degC
      settings: InternalSimscapePortConfiguration="{\"Bottom\":[],\"Left\":[{\"id\":\"A\",\"label\":\"A\",\"type\":\"foundation.thermal_liquid.thermal_liquid\"},{\"id\":\"C\",\"label\":\"C\",\"type\":\"foundation.mechanical.translational.translational\"},{\"id\":\"H\",\"label\":\"H\",\"type\":\"foundation.thermal.thermal\"}],\"Right\":[{\"id\":\"R\",\"label\":\"R\",\"type\":\"foundation.mechanical.translational.translational\"}],\"Top\":[]}"
  Mechanical Translational Reference : fl_lib/Mechanical/Translational Elements/Mechanical Translational Reference
  Perfect Insulator : fl_lib/Thermal/Thermal Elements/Perfect Insulator  T_specify=off  T_priority=None  T=0 K  T_nominal_specify=off  T_nominal_unit=K  T_nominal_value=1
  Translational Free End : fl_lib/Mechanical/Translational Elements/Translational Free End  v_specify=off  v_priority=None  v=0 m/s  v_nominal_specify=off  v_nominal_unit=m/s  v_nominal_value=1
      settings: InternalSimscapePortConfiguration="{\"Bottom\":[],\"Left\":[{\"id\":\"V\",\"label\":\"\",\"type\":\"foundation.mechanical.translational.translational\"}],\"Right\":[],\"Top\":[]}"
  T : PMIOPort  Side=Right
  connections:
  Perfect Insulator/LConn1 -- Coolant Volume/LConn3
  Translational Free End/LConn1 -- Coolant Volume/RConn1
  Mechanical Translational Reference/LConn1 -- Coolant Volume/LConn2
  Coolant Volume/LConn1 -- T/RConn1
